simulink model "Speedometer_Module"  (R2022a)
settings: Solver=FixedStepDiscrete  StartTime=0.0  StopTime=10.0  FixedStep=0.01  RelTol=1e-3
libraries: simulink x1
settings Model: DataDictionary=VSM_Data_Dictionary.sldd  EnableAccessToBaseWorkspace=off  DVExtractedSubsystem=Speedometer_Module  Creator=jamesbond  LastModifiedBy=jamesbond
settings OptimizationCC: DefaultParameterBehavior=Inlined  EnhancedBackFolding=on  PassReuseOutputArgsAs=Individual arguments  ZeroExternalMemoryAtStartup=off  ZeroInternalMemoryAtStartup=off  OptimizeBlockOrder=speed  DifferentSizesBufferReuse=on  OptimizationCustomize=off  EfficientTunableParamExpr=on
settings DebuggingCC: SignalInfNanChecking=error  SignalRangeChecking=warning  CheckMatrixSingularityMsg=error  IntegerOverflowMsg=none  ParameterOverflowMsg=none  ParameterTunabilityLossMsg=error  FrameProcessingCompatibilityMsg=none  BusObjectLabelMismatch=error  ModelReferenceVersionMismatchMessage=warning  ModelReferenceIOMismatchMessage=warning  IntegerSaturationMsg=none
settings SFSimCC: MATLABDynamicMemAlloc=off
settings RTWCC: SystemTargetFile=ert.tlc  TemplateMakefile=ert_default_tmf  GenerateReport=on
settings CodeAppCC: ForceParamTrailComments=on  IgnoreCustomStorageClasses=off  OperatorAnnotations=on  SimulinkDataObjDesc=on  SFDataObjDesc=on  InsertBlockDesc=on
settings ERTTargetCC: TargetLangStandard=C99 (ISO)  GenerateSampleERTMain=on  InlinedParameterPlacement=NonHierarchical  ERTCustomFileTemplate=example_file_process.tlc
settings ConfigComp: DVModelCoverageObjectives=MCDC  DVTestSuiteOptimization=Auto  DVDetectDeadLogic=on  DVDetectOutOfBounds=on  DVModelReferenceHarness=on  DVHarnessSource=Signal Editor

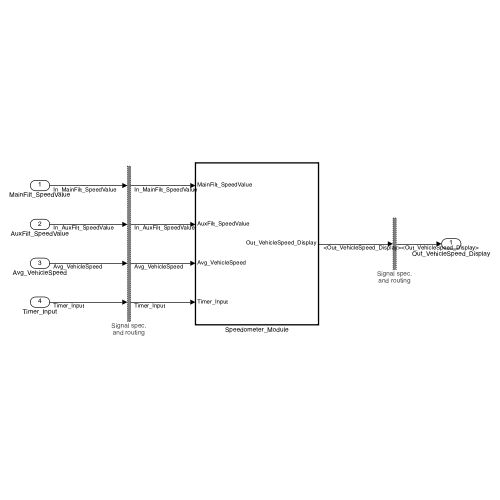
[thumbnail: Simulink's stored preview of the top-level diagram]
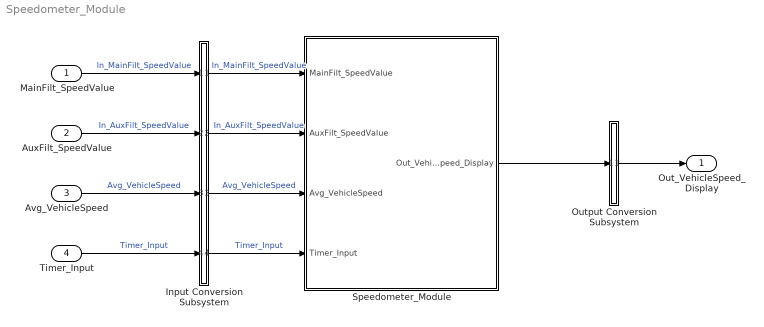
== system Speedometer_Module ==
  MainFilt_SpeedValue : Inport  OutMin=1  OutMax=3  OutDataTypeStr=uint8  PortDimensions=[1]  SampleTime=0.01  Interpolate=off
  AuxFilt_SpeedValue : Inport  Port=2  OutMin=1  OutMax=3  OutDataTypeStr=uint8  PortDimensions=[1]  SampleTime=0.01  Interpolate=off
  Avg_VehicleSpeed : Inport  Port=3  OutMin=0  OutMax=280  OutDataTypeStr=fixdt('ufix16_Sp01')  PortDimensions=[1]  SampleTime=0.01  Interpolate=off
  Timer_Input : Inport  Port=4  OutDataTypeStr=uint16  PortDimensions=[1]  SampleTime=0.01  Interpolate=off
  Input Conversion Subsystem : Subsystem  Tag=__SLT_ICS__  Description=|
      | Signal spec.
      | and routing
      settings: AttributesFormatString=%<Description>
  Output Conversion Subsystem : Subsystem  Tag=__SLT_OCS__  Description=|
      | Signal spec.
      | and routing
      settings: AttributesFormatString=%<Description>
  Speedometer_Module : Subsystem  TreatAsAtomicUnit=on
  Out_VehicleSpeed_Display : Outport
  wires:
  MainFilt_SpeedValue/1 -> Input Conversion Subsystem/1(Inport_1)  "In_MainFilt_SpeedValue"
  AuxFilt_SpeedValue/1 -> Input Conversion Subsystem/2(Inport_2)  "In_AuxFilt_SpeedValue"
  Avg_VehicleSpeed/1 -> Input Conversion Subsystem/3(Inport_3)  "Avg_VehicleSpeed"
  Timer_Input/1 -> Input Conversion Subsystem/4(Inport_4)  "Timer_Input"
  Output Conversion Subsystem/1(Outport_1) -> Out_VehicleSpeed_Display/1
  Input Conversion Subsystem/1(Outport_1) -> Speedometer_Module/1(MainFilt_SpeedValue)  "In_MainFilt_SpeedValue"
  Input Conversion Subsystem/2(Outport_2) -> Speedometer_Module/2(AuxFilt_SpeedValue)  "In_AuxFilt_SpeedValue"
  Input Conversion Subsystem/3(Outport_3) -> Speedometer_Module/3(Avg_VehicleSpeed)  "Avg_VehicleSpeed"
  Input Conversion Subsystem/4(Outport_4) -> Speedometer_Module/4(Timer_Input)  "Timer_Input"
  Speedometer_Module/1(Out_VehicleSpeed_Display) -> Output Conversion Subsystem/1(Inport_1)

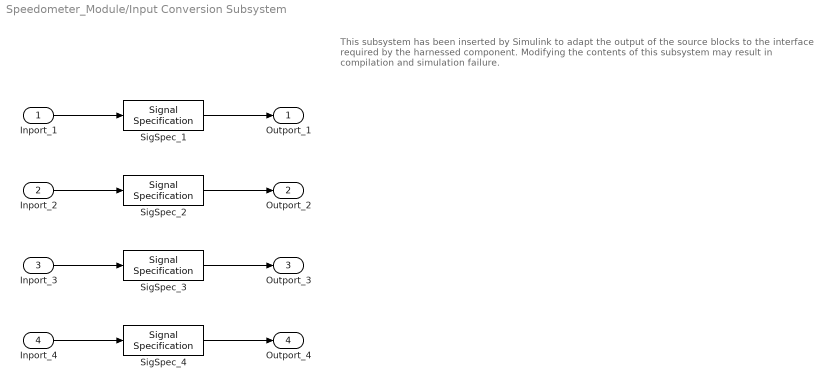
== system Speedometer_Module/Input Conversion Subsystem ==
  note: This subsystem has been inserted by Simulink to adapt the output of the source blocks to the interface required by the harnessed component.
      |  Modifying the contents of this subsystem may result in compilation and simulation failure.
  Inport_1 : Inport
  Inport_2 : Inport  Port=2
  Inport_3 : Inport  Port=3
  Inport_4 : Inport  Port=4
  SigSpec_1 : SignalSpecification  OutDataTypeStr=uint8  Dimensions=[1]  SampleTime=0.01
  SigSpec_2 : SignalSpecification  OutDataTypeStr=uint8  Dimensions=[1]  SampleTime=0.01
  SigSpec_3 : SignalSpecification  OutDataTypeStr=fixdt('ufix16_Sp01')  Dimensions=[1]  SampleTime=0.01
  SigSpec_4 : SignalSpecification  OutDataTypeStr=uint16  Dimensions=[1]  SampleTime=0.01
  Outport_1 : Outport
  Outport_2 : Outport  Port=2
  Outport_3 : Outport  Port=3
  Outport_4 : Outport  Port=4
  wires:
  SigSpec_1/1 -> Outport_1/1
  Inport_1/1 -> SigSpec_1/1
  SigSpec_2/1 -> Outport_2/1
  Inport_2/1 -> SigSpec_2/1
  SigSpec_3/1 -> Outport_3/1
  Inport_3/1 -> SigSpec_3/1
  SigSpec_4/1 -> Outport_4/1
  Inport_4/1 -> SigSpec_4/1

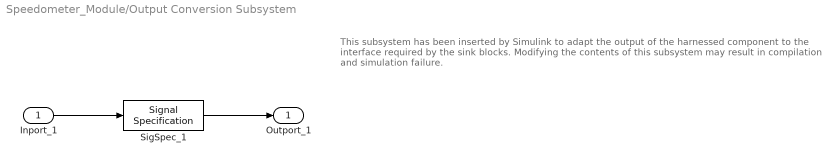
== system Speedometer_Module/Output Conversion Subsystem ==
  note: This subsystem has been inserted by Simulink to adapt the output of the harnessed component to the interface required by the sink blocks.
      |  Modifying the contents of this subsystem may result in compilation and simulation failure.
  Inport_1 : Inport
  SigSpec_1 : SignalSpecification  OutDataTypeStr=fixdt('ufix16_Sp01')  Dimensions=[1]  SampleTime=0.01
  Outport_1 : Outport
  wires:
  Inport_1/1 -> SigSpec_1/1
  SigSpec_1/1 -> Outport_1/1

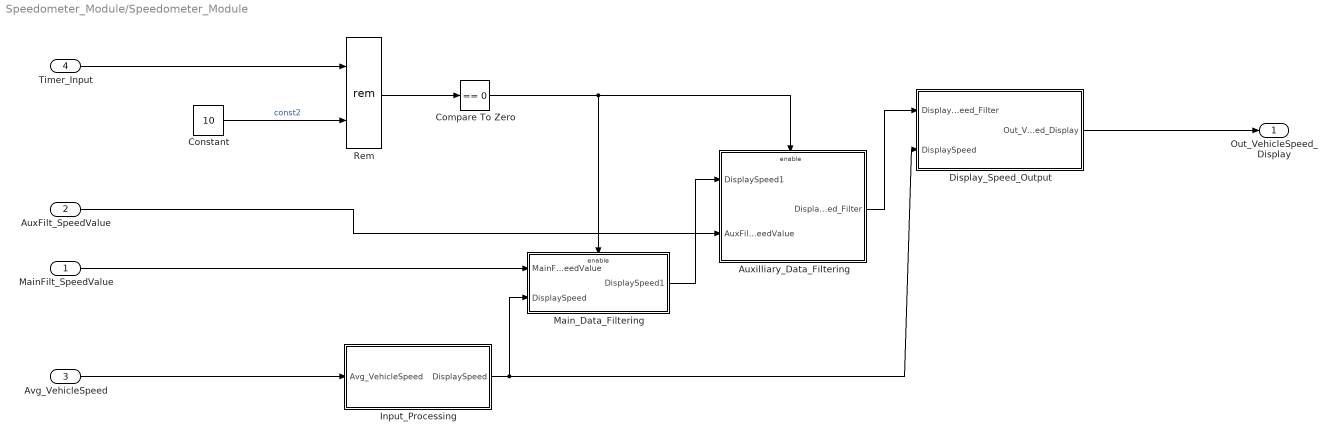
== system Speedometer_Module/Speedometer_Module ==
  MainFilt_SpeedValue : Inport  OutMin=1  OutMax=3  OutDataTypeStr=fixdt(0,8,1,0)  PortDimensions=1  SampleTime=0.01
  AuxFilt_SpeedValue : Inport  Port=2  OutMin=1  OutMax=3  OutDataTypeStr=fixdt(0,8,1,0)  PortDimensions=1  SampleTime=0.01
  Avg_VehicleSpeed : Inport  Port=3  OutMin=0  OutMax=280  OutDataTypeStr=fixdt(0,16,0.01,0)  PortDimensions=1  SampleTime=0.01
  Timer_Input : Inport  Port=4  OutDataTypeStr=fixdt(0,16,0)  PortDimensions=1  SampleTime=0.01
  Auxilliary_Data_Filtering : Subsystem
  Compare To Zero : simulink/Logic and Bit Operations/Compare To Zero  relop===  OutDataTypeStr=boolean
  Constant : Constant  Value=10  OutDataTypeStr=fixdt(0,16,0)
  Display_Speed_Output : Subsystem
  Input_Processing : Subsystem
  Main_Data_Filtering : Subsystem
  Rem : Math  Operator=rem
  Out_VehicleSpeed_Display : Outport
  wires:
  AuxFilt_SpeedValue/1 -> Auxilliary_Data_Filtering/2(AuxFilt_SpeedValue)
  Main_Data_Filtering/1(DisplaySpeed1) -> Auxilliary_Data_Filtering/1(DisplaySpeed1)
  Compare To Zero/1 -> Auxilliary_Data_Filtering/Enable, Main_Data_Filtering/Enable
  Rem/1 -> Compare To Zero/1
  Constant/1 -> Rem/2  "const2"
  Timer_Input/1 -> Rem/1
  Display_Speed_Output/1(Out_VehicleSpeed_Display) -> Out_VehicleSpeed_Display/1
  Auxilliary_Data_Filtering/1(DisplaySpeed_Filter) -> Display_Speed_Output/1(DisplaySpeed_Filter)
  Input_Processing/1(DisplaySpeed) -> Display_Speed_Output/2(DisplaySpeed), Main_Data_Filtering/2(DisplaySpeed)
  MainFilt_SpeedValue/1 -> Main_Data_Filtering/1(MainFilt_SpeedValue)
  Avg_VehicleSpeed/1 -> Input_Processing/1(Avg_VehicleSpeed)

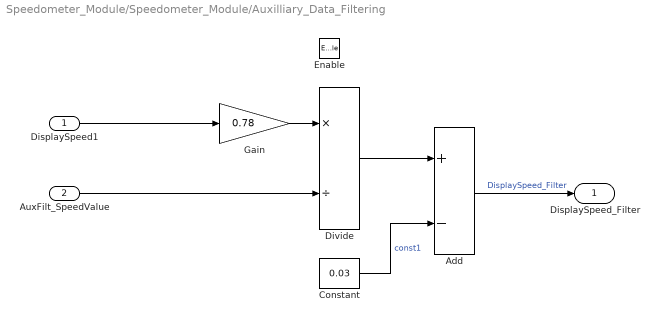
== system Speedometer_Module/Speedometer_Module/Auxilliary_Data_Filtering ==
  DisplaySpeed1 : Inport  OutDataTypeStr=fixdt(0,16,0.01,0)  PortDimensions=1  SampleTime=0.01
  AuxFilt_SpeedValue : Inport  Port=2
  Enable : EnablePort
  Add : Sum  Inputs=+-  AccumDataTypeStr=fixdt(0,16,0.01,0)  OutDataTypeStr=fixdt(0,16,0.01,0)
  Constant : Constant  Value=0.03  OutMin=0.03  OutMax=0.03  OutDataTypeStr=fixdt(0,16,0.01,0)
  Divide : Product  Inputs=*/  OutDataTypeStr=fixdt(0,16,0.01,0)
  Gain : Gain  Gain=0.78  ParamMin=0.78  ParamMax=0.78  ParamDataTypeStr=fixdt(0,16,0.01,0)  OutDataTypeStr=fixdt(0,16,0.01,0)
  DisplaySpeed_Filter : Outport  OutDataTypeStr=fixdt(0,16,0.01,0)  PortDimensions=1  SampleTime=0.01
  wires:
  Divide/1 -> Add/1
  AuxFilt_SpeedValue/1 -> Divide/2
  DisplaySpeed1/1 -> Gain/1
  Constant/1 -> Add/2  "const1"
  Add/1 -> DisplaySpeed_Filter/1  "DisplaySpeed_Filter"
  Gain/1 -> Divide/1

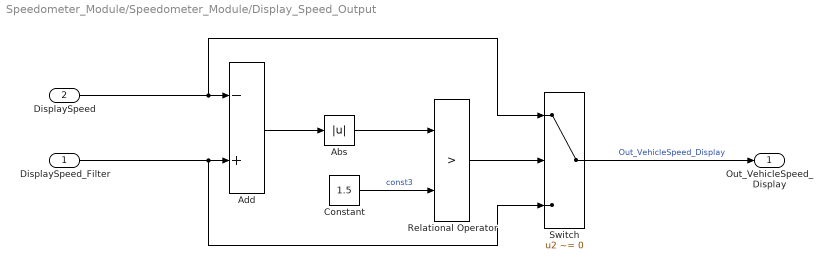
== system Speedometer_Module/Speedometer_Module/Display_Speed_Output ==
  DisplaySpeed_Filter : Inport  OutDataTypeStr=fixdt(0,16,0.01,0)  PortDimensions=1  SampleTime=0.01
  DisplaySpeed : Inport  Port=2  OutDataTypeStr=fixdt(0,16,0.01,0)  PortDimensions=1  SampleTime=0.01
  Abs : Abs  OutDataTypeStr=fixdt(0,16,0.01,0)  SaturateOnIntegerOverflow=off
  Add : Sum  Inputs=-+  AccumDataTypeStr=fixdt(0,16,0.01,0)  OutDataTypeStr=fixdt(0,16,0.01,0)
  Constant : Constant  Value=1.5  OutMin=1.5  OutMax=1.5  OutDataTypeStr=fixdt(0,16,0.01,0)
  Relational Operator : RelationalOperator  Operator=>  OutDataTypeStr=boolean  RndMeth=Simplest  InputSameDT=off
  Switch : Switch  Criteria=u2 ~= 0  OutDataTypeStr=fixdt(0,16,0.01,0)  SaturateOnIntegerOverflow=off  InputSameDT=off
  Out_VehicleSpeed_Display : Outport
  wires:
  Switch/1 -> Out_VehicleSpeed_Display/1  "Out_VehicleSpeed_Display"
  Relational Operator/1 -> Switch/2
  Constant/1 -> Relational Operator/2  "const3"
  Abs/1 -> Relational Operator/1
  Add/1 -> Abs/1
  DisplaySpeed_Filter/1 -> Switch/3, Add/2
  DisplaySpeed/1 -> Add/1, Switch/1

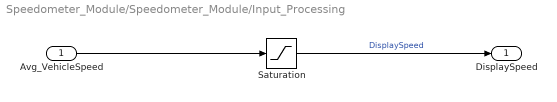
== system Speedometer_Module/Speedometer_Module/Input_Processing ==
  Avg_VehicleSpeed : Inport  OutMin=0  OutMax=280  OutDataTypeStr=fixdt(0,16,0.01,0)  PortDimensions=1  SampleTime=0.01
  Saturation : Saturate  UpperLimit=250  LowerLimit=2  OutDataTypeStr=fixdt(0,16,0.01,0)
  DisplaySpeed : Outport  OutDataTypeStr=fixdt(0,16,0.01,0)  PortDimensions=1  SampleTime=0.01
  wires:
  Avg_VehicleSpeed/1 -> Saturation/1
  Saturation/1 -> DisplaySpeed/1  "DisplaySpeed"

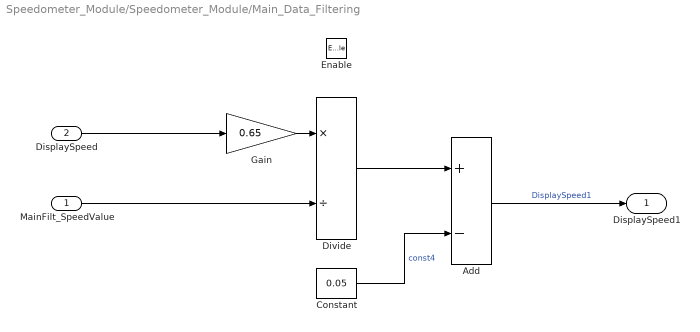
== system Speedometer_Module/Speedometer_Module/Main_Data_Filtering ==
  MainFilt_SpeedValue : Inport  OutMin=1  OutMax=3  OutDataTypeStr=fixdt(0,8,1,0)  PortDimensions=1  SampleTime=0.01
  DisplaySpeed : Inport  Port=2  OutDataTypeStr=fixdt(0,16,0.01,0)  PortDimensions=1  SampleTime=0.01
  Enable : EnablePort
  Add : Sum  Inputs=+-  AccumDataTypeStr=fixdt(0,16,0.01,0)  OutDataTypeStr=fixdt(0,16,0.01,0)
  Constant : Constant  Value=0.05  OutMin=0.05  OutMax=0.05  OutDataTypeStr=fixdt(0,16,0.01,0)
  Divide : Product  Inputs=*/  OutDataTypeStr=fixdt(0,16,0.01,0)
  Gain : Gain  Gain=0.65  ParamMin=0.65  ParamMax=0.65  ParamDataTypeStr=fixdt(0,16,0.01,0)  OutDataTypeStr=fixdt(0,16,0.01,0)
  DisplaySpeed1 : Outport  OutDataTypeStr=fixdt(0,16,0.01,0)  PortDimensions=1  SampleTime=0.01
  wires:
  MainFilt_SpeedValue/1 -> Divide/2
  DisplaySpeed/1 -> Gain/1
  Constant/1 -> Add/2  "const4"
  Add/1 -> DisplaySpeed1/1  "DisplaySpeed1"
  Divide/1 -> Add/1
  Gain/1 -> Divide/1
